simulink library "pathProjectionWithWarping_ul"  (R2018a)
settings: Solver=VariableStepAuto  StartTime=0.0  StopTime=10.0  RelTol=1e-3
values from neighbouring files (symbols this model uses):
  pathHeight_m = 10    [pathProjectionWithWarping_ts.m]
  pathWidth_m = 100    [pathProjectionWithWarping_ts.m]
  searchDistance_none = 0.2    [pathProjectionWithWarping_init.m]
  warpingFactor_none = -0.8    [pathProjectionWithWarping_ts.m]
settings Model: Creator=mcobb  LastModifiedBy=mcobb

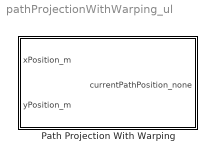
== system pathProjectionWithWarping_ul ==
  Path Projection With Warping : Subsystem

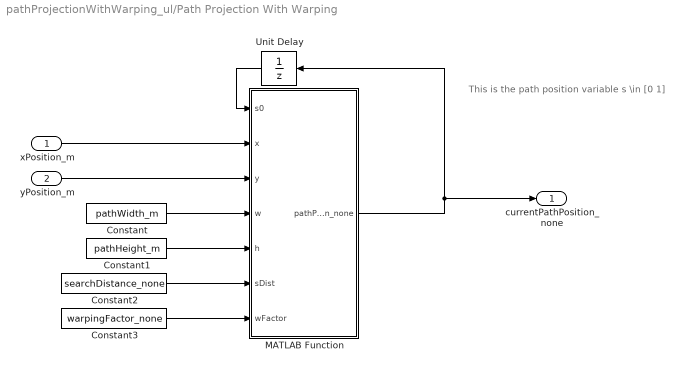
== system pathProjectionWithWarping_ul/Path Projection With Warping ==
  note: This is the path position variable s \in [0 1]
  xPosition_m : Inport
  yPosition_m : Inport  Port=2
  Constant : Constant  Value=pathWidth_m
  Constant1 : Constant  Value=pathHeight_m
  Constant2 : Constant  Value=searchDistance_none
  Constant3 : Constant  Value=warpingFactor_none
  MATLAB Function : MATLAB Function  TreatAsAtomicUnit=on
  Unit Delay : UnitDelay  SampleTime=-1
  currentPathPosition_none : Outport
  wires:
  Unit Delay/1 -> MATLAB Function/1(s0)
  xPosition_m/1 -> MATLAB Function/2(x)
  yPosition_m/1 -> MATLAB Function/3(y)
  Constant/1 -> MATLAB Function/4(w)
  Constant1/1 -> MATLAB Function/5(h)
  Constant2/1 -> MATLAB Function/6(sDist)
  MATLAB Function/1(pathPosition_none) -> Unit Delay/1, currentPathPosition_none/1
  Constant3/1 -> MATLAB Function/7(wFactor)

== matlab function pathProjectionWithWarping_ul/Path Projection With Warping/MATLAB Function ==
  data: s0 input; pathPosition_none output; x input; y input; w input; h input; sDist input; wFactor input
function pathPosition_none = fcn(s0,x,y,w,h,sDist,wFactor)
pathPosition_none = pathProjectionWithWarping(s0,x,y,w,h,sDist,wFactor);
end
